simulink model "fig656d"  (Simulink 3.00)
settings: Solver=ode45  SolverMode=SingleTasking  StartTime=0.0  StopTime=2  RelTol=1e-3  AbsTol=1e-6
libraries: simulink3 x3

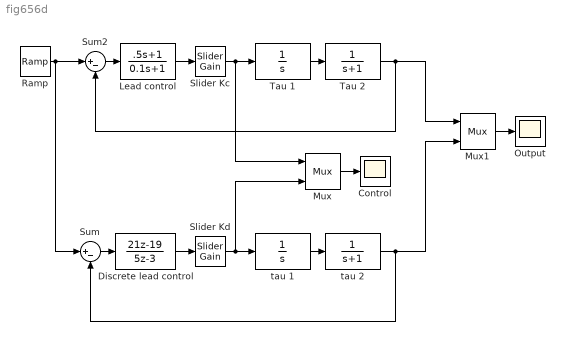
== system fig656d ==
  Control : Scope
      settings: TickLabels=on  TimeRange=auto  YMin=0  YMax=2.75  SaveName=ucd  DataFormat=Matrix
  Discrete lead control : DiscreteTransferFcn  Numerator=[21 -19]  Denominator=[5 -3]  SampleTime=.05
  Lead control : TransferFcn  Numerator=[.5 1]  Denominator=[0.1 1]
  Mux : Mux  Inputs=2
      settings: DisplayOption=none
  Mux1 : Mux  Inputs=2
      settings: DisplayOption=none
  Output : Scope
      settings: TickLabels=on  TimeRange=auto  YMin=-5  YMax=5  SaveName=ycd  DataFormat=Matrix
  Ramp : simulink3/Sources/Ramp  slope=1  start=0  X0=0
  Slider Kc : simulink3/Math/Slider Gain  low=0  gain=10  high=20
  Slider Kd : simulink3/Math/Slider Gain  low=0  gain=10  high=20
  Sum : Sum  Inputs=|+-  SaturateOnIntegerOverflow=off
  Sum2 : Sum  Inputs=|+-  SaturateOnIntegerOverflow=off
  Tau 1 : TransferFcn  Numerator=1  Denominator=[1 0]
  Tau 2 : TransferFcn  Numerator=1  Denominator=[1 1]
  tau 1 : TransferFcn  Numerator=1  Denominator=[1 0]
  tau 2 : TransferFcn  Numerator=1  Denominator=[1 1]
  wires:
  Lead control/1 -> Slider Kc/1
  Sum2/1 -> Lead control/1
  Tau 1/1 -> Tau 2/1
  Discrete lead control/1 -> Slider Kd/1
  tau 1/1 -> tau 2/1
  Ramp/1 -> Sum2/1, Sum/1
  Slider Kc/1 -> Tau 1/1, Mux/1
  Mux/1 -> Control/1
  Tau 2/1 -> Mux1/1, Sum2/2
  Mux1/1 -> Output/1
  Sum/1 -> Discrete lead control/1
  Slider Kd/1 -> tau 1/1, Mux/2
  tau 2/1 -> Mux1/2, Sum/2
